simulink model "template_matching_plus_sd"  (R2019b)
settings: Solver=VariableStepAuto  StartTime=0.0  StopTime=10  RelTol=1e-3
libraries: simulink x3, hdlsllib x1
settings Model: Creator=sbuccelli  LastModifiedBy=sbuccelli

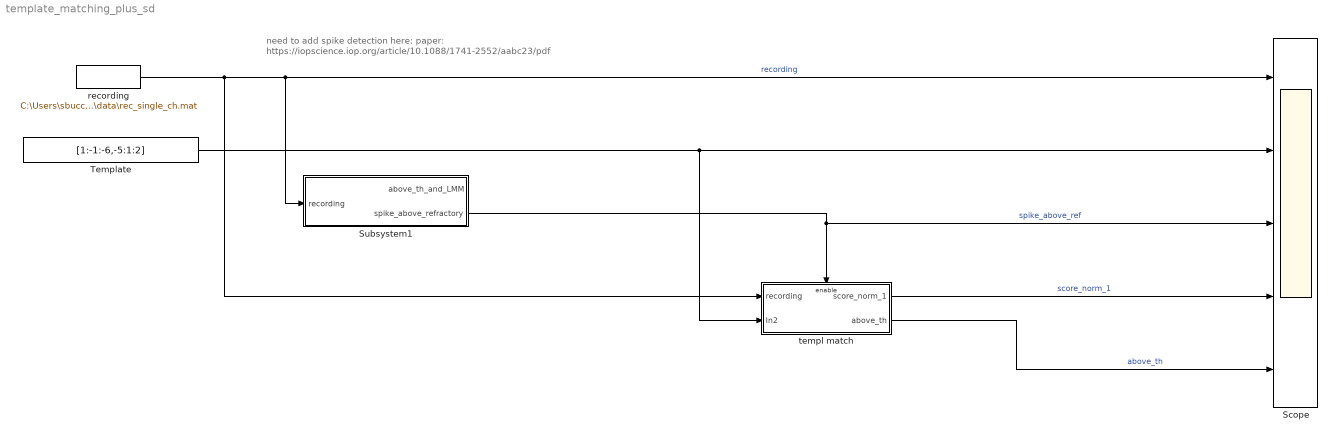
== system template_matching_plus_sd ==
  note: need to add spike detection here:
      | paper: https://iopscience.iop.org/article/10.1088/1741-2552/aabc23/pdf
  Scope : Scope  NumInputPorts=5
  Subsystem1 : Subsystem
  Template : Constant  Value=[1:-1:-6,-5:1:2]  SampleTime=-1
  recording : FromFile  FileName=C:\Users\sbuccelli\Documents\GitHub\closed-loop-neuroscience\data\rec_single_ch.mat  SampleTime=1/32e3
  templ match : Subsystem
  wires:
  Template/1 -> templ match/2(In2), Scope/2
  recording/1 -> templ match/1(recording), Scope/1, Subsystem1/1(recording)  "recording"
  templ match/1(score_norm_1) -> Scope/4  "score_norm_1"
  templ match/2(above_th) -> Scope/5  "above_th"
  Subsystem1/2(spike_above_refractory) -> Scope/3, templ match/Enable  "spike_above_ref"

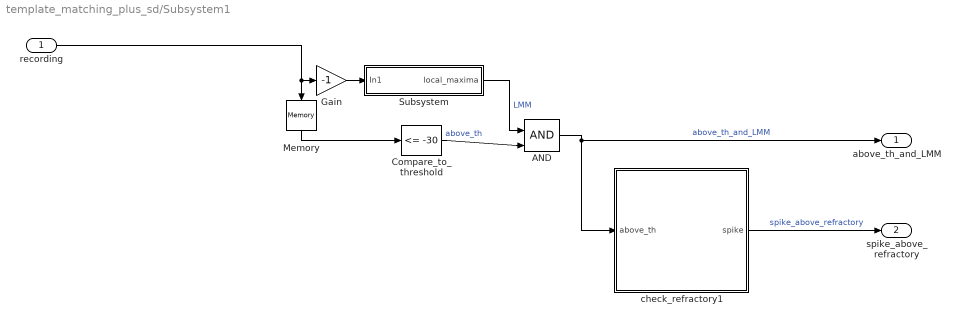
== system template_matching_plus_sd/Subsystem1 ==
  recording : Inport
  AND : Logic  IconShape=distinctive  AllPortsSameDT=off  OutDataTypeStr=boolean
  Compare_to_threshold : simulink/Logic and Bit Operations/Compare To Constant  relop=<=  const=-30  OutDataTypeStr=boolean
  Gain : Gain  Gain=-1
  Memory : Memory  InheritSampleTime=on
  Subsystem : Subsystem
  check_refractory1 : Subsystem
  above_th_and_LMM : Outport
  spike_above_refractory : Outport  Port=2
  wires:
  recording/1 -> Memory/1, Gain/1
  check_refractory1/1(spike) -> spike_above_refractory/1  "spike_above_refractory"
  AND/1 -> above_th_and_LMM/1, check_refractory1/1(above_th)  "above_th_and_LMM"
  Subsystem/1(local_maxima) -> AND/1  "LMM"
  Gain/1 -> Subsystem/1(In1)
  Compare_to_threshold/1 -> AND/2  "above_th"
  Memory/1 -> Compare_to_threshold/1

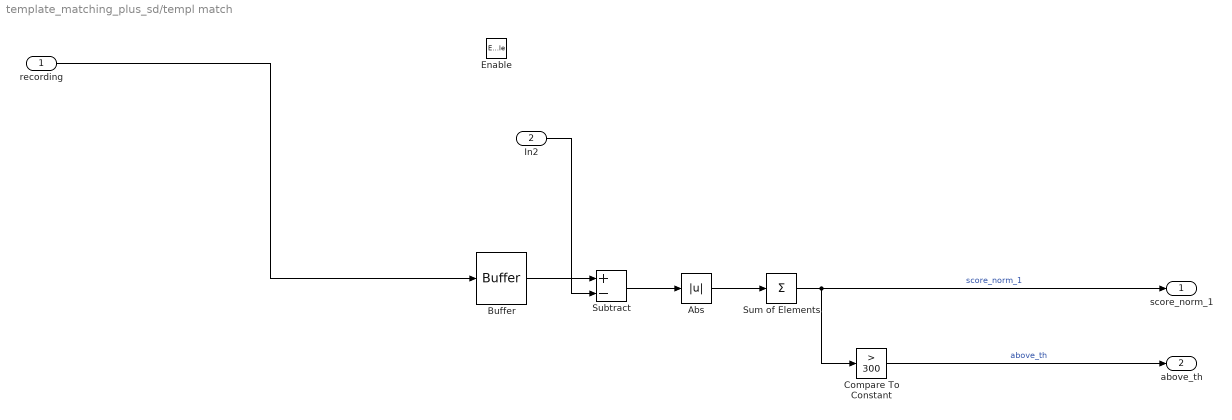
== system template_matching_plus_sd/templ match ==
  recording : Inport
  In2 : Inport  Port=2
  Enable : EnablePort
  Abs : Abs
  Buffer : Buffer  N=16  V=15  OutputFrames=off
  Compare To Constant : simulink/Logic and Bit Operations/Compare To Constant  relop=>  const=300  OutDataTypeStr=boolean
  Subtract : Sum  Inputs=+-
  Sum of Elements : Sum  Inputs=+
  score_norm_1 : Outport  OutputWhenDisabled=reset  InitialOutput=0
  above_th : Outport  Port=2  OutputWhenDisabled=reset  InitialOutput=0
  wires:
  Compare To Constant/1 -> above_th/1  "above_th"
  Buffer/1 -> Subtract/1
  Sum of Elements/1 -> score_norm_1/1, Compare To Constant/1  "score_norm_1"
  Subtract/1 -> Abs/1
  In2/1 -> Subtract/2
  recording/1 -> Buffer/1
  Abs/1 -> Sum of Elements/1

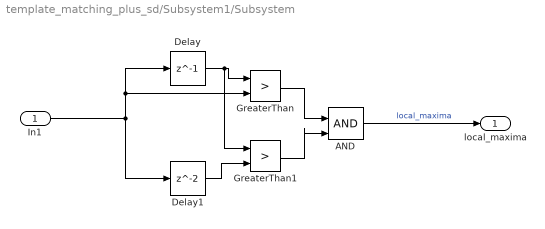
== system template_matching_plus_sd/Subsystem1/Subsystem ==
  In1 : Inport
  AND : Logic  IconShape=distinctive  AllPortsSameDT=off  OutDataTypeStr=boolean
  Delay : Delay  DelayLength=1
  Delay1 : Delay
  GreaterThan : RelationalOperator  Operator=>  OutDataTypeStr=boolean  RndMeth=Simplest
  GreaterThan1 : RelationalOperator  Operator=>  OutDataTypeStr=boolean  RndMeth=Simplest
  local_maxima : Outport
  wires:
  Delay1/1 -> GreaterThan1/2
  GreaterThan1/1 -> AND/2
  GreaterThan/1 -> AND/1
  Delay/1 -> GreaterThan1/1, GreaterThan/1
  AND/1 -> local_maxima/1  "local_maxima"
  In1/1 -> Delay/1, GreaterThan/2, Delay1/1

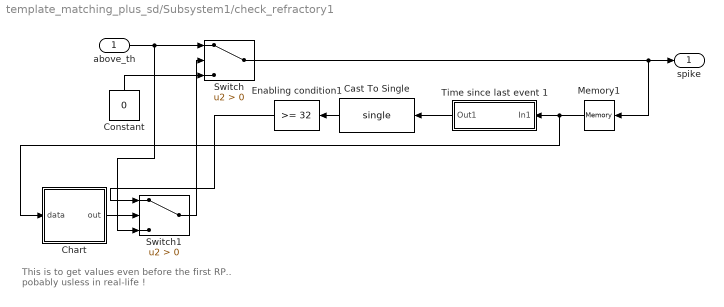
== system template_matching_plus_sd/Subsystem1/check_refractory1 ==
  note: This is to get values even before the first RP.. pobably usless in real-life !
  above_th : Inport
  Cast To Single : DataTypeConversion  OutDataTypeStr=single
  Chart : Stateflow chart  BlockKeywords=__PRM__SERIALIZED__DATA__:Stateflow Chart,Stateflow Diagram  TreatAsAtomicUnit=on
  Constant : Constant  Value=0  OutDataTypeStr=boolean
  Enabling condition1 : simulink/Logic and Bit Operations/Compare To Constant  relop=>=  const=32  OutDataTypeStr=boolean
  Memory1 : Memory  InheritSampleTime=on
  Switch : Switch  Criteria=u2 > Threshold
  Switch1 : Switch  Criteria=u2 > Threshold
  Time since last event 1 : Subsystem
  spike : Outport
  wires:
  Switch/1 -> spike/1, Memory1/1
  above_th/1 -> Switch1/3, Switch/1
  Memory1/1 -> Chart/1(data), Time since last event 1/1(In1)
  Time since last event 1/1(Out1) -> Cast To Single/1
  Enabling condition1/1 -> Switch1/1
  Constant/1 -> Switch/3
  Cast To Single/1 -> Enabling condition1/1
  Chart/1(out) -> Switch1/2
  Switch1/1 -> Switch/2

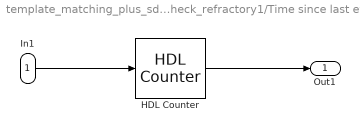
== system template_matching_plus_sd/Subsystem1/check_refractory1/Time since last event 1 ==
  In1 : Inport
  HDL Counter : hdlsllib/Sources/HDL Counter  CountType=Free running  CountInit=1  CountStep=1  CountMax=25  CountFromType=Initial value  CountFrom=1  CountResetPort=on  CountLoadPort=off  CountEnbPort=off  CountDirPort=off  CountDataType=Unsigned  CountWordLen=32  CountFracLen=0  CountSampTime=1
      settings: SourceProductName=Simulink
  Out1 : Outport
  wires:
  In1/1 -> HDL Counter/1
  HDL Counter/1 -> Out1/1

== stateflow chart template_matching_plus_sd/Subsystem1/check_refractory1/Chart ==
  settings: stateMachineType=MOORE_MACHINE
  state zero
    out=0
  state zero1
    out=1
  (default) -> zero
  zero -> zero1 : [data==1]
  data: data input; out output
